simulink model "EarlyReturn7"  (R2020b)
settings: Solver=VariableStepAuto  StartTime=0.0  StopTime=0.2  RelTol=1e-3
settings Model: Creator=BEAR  LastModifiedBy=apple
settings DataIOCC: ReturnWorkspaceOutputs=off
settings DebuggingCC: ArithmeticOperatorsInVariantConditions=warning
settings SFSimCC: SimUseLocalCustomCode=off  CustomCodeUndefinedFunction=UseInterfaceOnly
settings RTWCC: RTWUseLocalCustomCode=off

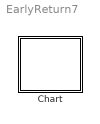
== system EarlyReturn7 ==
  Chart : Stateflow chart  TreatAsAtomicUnit=on

== stateflow chart EarlyReturn7/Chart ==
  settings: updateMethod=DISCRETE  sampleTime=0.1
  state A
    en: fprintf("en_A")
    ex: fprintf("ex_A")
    state A1
      en: fprintf("en_A1")
      ex: fprintf("ex_A1")
    state A2
      en: fprintf("en_A2")
      ex: fprintf("ex_A2")
    state A3
      en: fprintf("en_A3")
      ex: fprintf("ex_A3")
    (default) -> A1
    A1 -> A2
    A2 -> A3 : /{E;fprintf("ta")}
  (default) -> A
  A -> A : E{fprintf("loop")}
  events: E local FUNCTION_CALL_EVENT
